simulink model "Iterative_Inverse_Kinematics"  (R2024a)
settings: Solver=ode4  StartTime=0.0  StopTime=inf  FixedStep=1/500  RelTol=1e-3  EnableMultiTasking=on
InitFcn:
  | home = [0.45; 0; 0.49];
  | default_w = [0.25; 0.25; 0.25];
  | default_a = [0.00; 0.375; 0.2];
  | A = [ 0.25; 0.25; 0.1];
  | B = [ 0.25; 0.50; 0.1];
  | C = [-0.25; 0.50; 0.1];
  | D = [-0.25; 0.25; 0.1];
  | 
  | waypoints_welding = [default_w, A, B, C, D, A]' ;
  | waypoints_assembly = [default_a, A, default_a, B, default_a, C, default_a, D]' ;
  | 
  | waypoints = waypoints_welding;
undefined symbols (not defined in the file): HIL, qc_get_step_size
libraries: quarc_library x9, simulink x2
settings Model: SimulationMode=external  ExtModeTrigDuration=10000  Creator=fvranes  LastModifiedBy=mbohra
settings SolverCC: AlgebraicLoopSolver=TrustRegion  PositivePriorityOrder=on
settings DataIOCC: SaveOutput=off  SignalLogging=off  DSMLogging=off  SaveTime=off  ReturnWorkspaceOutputs=off
settings DebuggingCC: UnconnectedInputMsg=warning  UnconnectedOutputMsg=warning  UnconnectedLineMsg=warning  ArithmeticOperatorsInVariantConditions=warning
settings ModelReferenceCC: EnableRefExpFcnMdlSchedulingChecks=on
settings SFSimCC: SimUseLocalCustomCode=off  CustomCodeUndefinedFunction=UseInterfaceOnly
settings RTWCC: Description=QUARC Win64 Target Using Toolchain  SystemTargetFile=quarc_win64.tlc  TemplateMakefile=quarc_default_tmf  RTWUseLocalCustomCode=off  Toolchain=QUARC win64 | nmake (64-bit Windows)  BuildConfiguration=Faster Runs  GPUComputeCapability=3.5
settings CodeAppCC: StateflowObjectComments=on
settings STFCustomTargetCC: ConcurrentExecutionCompliant=on  SystemTargetFile=quarc_win64.tlc
settings GRTTargetCC: ParMdlRefBuildCompliant=off  CompOptLevelCompliant=off  CombineOutputUpdateFcns=off  MatFileLogging=off  CPPClassGenCompliant=off  GRTInterface=on  ExtMode=on  ExtModeMexFile=quarc_comm
settings ConfigComp: CovMetricSettings=dswe

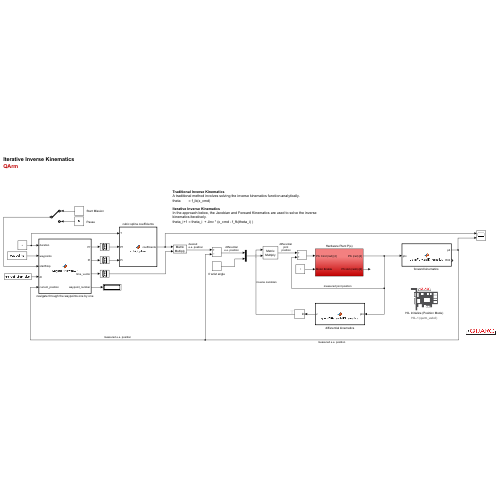
[thumbnail: Simulink's stored preview of the top-level diagram]
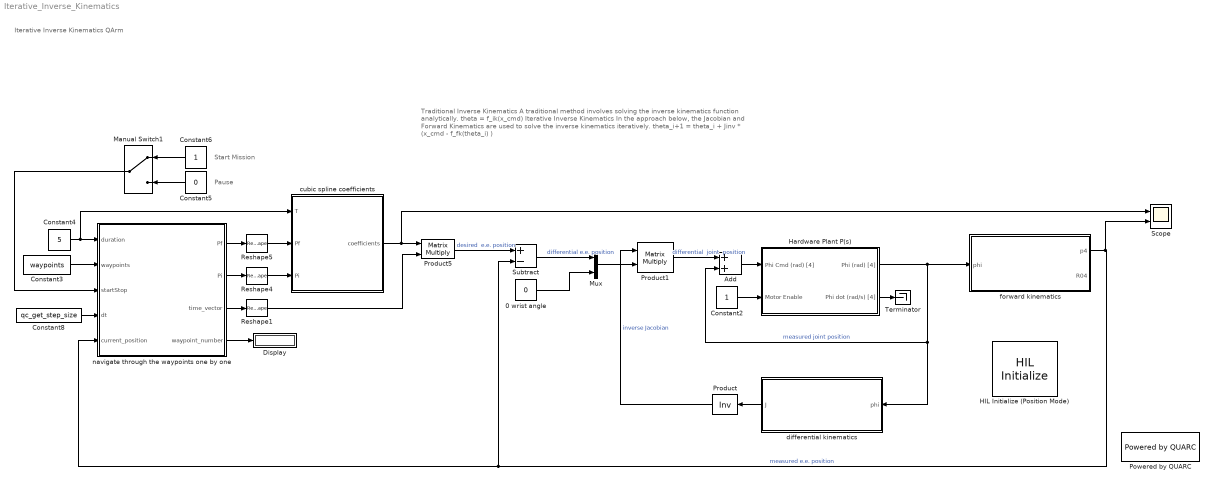
== system Iterative_Inverse_Kinematics ==
  note: Traditional Inverse Kinematics
      | A traditional method involves solving the inverse kinematics function analytically.
      | theta = f_ik(x_cmd)
      |
      | Iterative Inverse Kinematics
      | In the approach below, the Jacobian and Forward Kinematics are used to solve the inverse kinematics iteratively.
      | theta_i+1 = theta_i + Jinv * (x_cmd - f_fk(theta_i) )
  note: Iterative Inverse Kinematics
      | QArm
  note: Pause
  note: Start Mission
  0 wrist angle : Constant  Value=0
  Add : Sum
  Constant2 : Constant
  Constant3 : Constant  Value=waypoints  VectorParams1D=off
  Constant4 : Constant  Value=5
  Constant5 : Constant  Value=0
  Constant6 : Constant
  Constant8 : Constant  Value=qc_get_step_size
  Display : Display
  HIL Initialize (Position Mode) : quarc_library/Data Acquisition/Generic/Configuration/HIL Initialize  Priority=1  object_name=HIL-1  board_type=qarm_usb  board_number=0  board_options=j0_mode=0;j1_mode=0;j2_mode=0;j3_mode=0;gripper_mode=0;j0_profile_config=0;j0_profile_velocity=0;j0_profile_acceleration=0;j1_profile_config=0;j1_profile_velocity=0;j1_profile_acceleration=0;j2_profile_config=0;j2_profile_velocity=0;j2_profile_acceleration=0;j3_profile_config=0;j3_profile_velocity=0;j3_profile_acceleration=0;  exclusive=off  active=on  hardware_clocks=[0]  clock_modes=[]  initial_clock_frequencies=[]  set_clock_params_at_start=off  set_clock_params_at_switch_in=off  set_clock_frequencies_at_start=off  set_clock_frequencies_at_switch_in=off  analog_input_channels=[5:9]  analog_input_configurations=[]  analog_input_maximums=[]  analog_input_minimums=[]  set_analog_input_params_at_start=off  set_analog_input_params_at_switch_in=off  analog_output_channels=[]  analog_output_maximums=inf  analog_output_minimums=-inf  initial_analog_outputs=[0]  final_analog_outputs=[0]  watchdog_analog_outputs=[]  set_analog_output_params_at_start=off  set_analog_output_params_at_switch_in=off  set_analog_outputs_at_start=off  set_analog_outputs_at_switch_in=off  set_analog_outputs_at_terminate=off  set_analog_outputs_at_switch_out=off  set_analog_outputs_on_watchdog=off  digital_input_channels=[]  digital_output_channels=[]  digital_output_configuration=[]  initial_digital_outputs=[0]  final_digital_outputs=[0]  watchdog_digital_outputs=[0]  set_digital_output_params_at_start=off  set_digital_output_params_at_switch_in=off  set_digital_outputs_at_start=off  set_digital_outputs_at_switch_in=off  set_digital_outputs_at_terminate=off  set_digital_outputs_at_switch_out=off  set_digital_outputs_on_watchdog=off  encoder_channels=[]  quadrature=[]  encoder_filter_frequency=[]  initial_encoder_counts=[]  set_encoder_params_at_start=off  set_encoder_params_at_switch_in=off  set_encoder_counts_at_start=off  set_encoder_counts_at_switch_in=off  pwm_channels=[]  pwm_modes=[]  pwm_frequency=[]  pwm_configuration=[]  pwm_alignment=[]  pwm_polarity=[]  pwm_leading_deadband=[]  pwm_trailing_deadband=[]  initial_pwm_outputs=[]  final_pwm_outputs=[]  watchdog_pwm_outputs=[]  set_pwm_params_at_start=off  set_pwm_params_at_switch_in=off  set_pwm_outputs_at_start=off  set_pwm_outputs_at_switch_in=off  set_pwm_outputs_at_terminate=off  set_pwm_outputs_at_switch_out=off  set_pwm_outputs_on_watchdog=off  other_output_channels=[1000:1004 11000:11003 11005:11007]  initial_other_outputs=[zeros(1,9), ones(1,3)]  final_other_outputs=[zeros(1,9), ones(1,3)]  watchdog_other_outputs=zeros(1,12)  set_other_outputs_at_start=off  set_other_outputs_at_switch_in=off  set_other_outputs_at_terminate=off  set_other_outputs_at_switch_out=off  set_other_outputs_on_watchdog=off
  Hardware Plant P(s) : Subsystem
  Manual Switch1 : ManualSwitch
  Mux : Mux  Inputs=2
  Powered by QUARC : quarc_library/Logos/Powered by QUARC
  Product : Product  Inputs=/  Multiplication=Matrix(*)
  Product1 : Product  Multiplication=Matrix(*)
  Product5 : Product  Multiplication=Matrix(*)
  Reshape1 : Reshape  OutputDimensionality=Column vector (2-D)
  Reshape4 : Reshape  OutputDimensionality=Column vector (2-D)
  Reshape5 : Reshape  OutputDimensionality=Column vector (2-D)
  Scope : Scope  NumInputPorts=2
  Subtract : Sum  Inputs=+-
  Terminator : Terminator
  cubic spline coefficients : MATLAB Function  TreatAsAtomicUnit=on
  differential kinematics : MATLAB Function  TreatAsAtomicUnit=on
  "forward kinematics " : MATLAB Function  TreatAsAtomicUnit=on
  navigate through the waypoints one by one : MATLAB Function  TreatAsAtomicUnit=on
  wires:
  differential kinematics/1(J) -> Product/1
  Hardware Plant P(s)/1(Phi (rad) [4]) -> differential kinematics/1(phi), Add/2, "forward kinematics "/1(phi)  "measured joint position"
  "forward kinematics "/1(p4) -> Scope/2, navigate through the waypoints one by one/5(current_position), Subtract/2  "measured e.e. position"
  Product5/1 -> Subtract/1  "desired  e.e. position"
  Subtract/1 -> Mux/1  "differential e.e. position"
  Product/1 -> Product1/1  "inverse Jacobian"
  0 wrist angle/1 -> Mux/2
  Mux/1 -> Product1/2
  Product1/1 -> Add/1  "differential  joint  position"
  Add/1 -> Hardware Plant P(s)/1(Phi Cmd (rad) [4])
  Constant2/1 -> Hardware Plant P(s)/2(Motor Enable)
  Hardware Plant P(s)/2(Phi dot (rad/s) [4]) -> Terminator/1
  Reshape5/1 -> cubic spline coefficients/2(Pf)
  Constant5/1 -> Manual Switch1/2
  navigate through the waypoints one by one/3(time_vector) -> Reshape1/1
  Constant3/1 -> navigate through the waypoints one by one/2(waypoints)
  Reshape1/1 -> Product5/2
  Constant8/1 -> navigate through the waypoints one by one/4(dt)
  Constant4/1 -> cubic spline coefficients/1(T), navigate through the waypoints one by one/1(duration)
  navigate through the waypoints one by one/1(Pf) -> Reshape5/1
  Manual Switch1/1 -> navigate through the waypoints one by one/3(startStop)
  navigate through the waypoints one by one/2(Pi) -> Reshape4/1
  cubic spline coefficients/1(coefficients) -> Scope/1, Product5/1
  Constant6/1 -> Manual Switch1/1
  navigate through the waypoints one by one/4(waypoint_number) -> Display/1
  Reshape4/1 -> cubic spline coefficients/3(Pi)

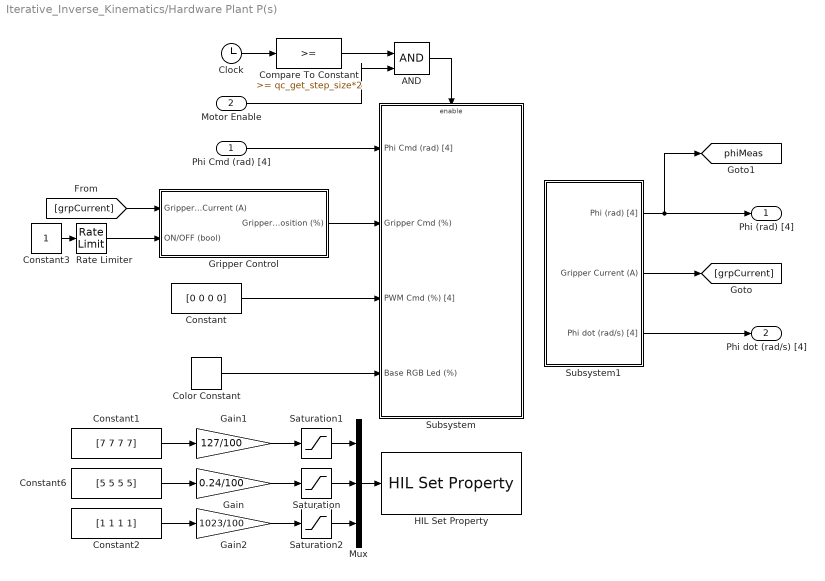
== system Iterative_Inverse_Kinematics/Hardware Plant P(s) ==
  Phi Cmd (rad) [4] : Inport
  Motor Enable : Inport  Port=2
  AND : Logic  IconShape=distinctive  AllPortsSameDT=off  OutDataTypeStr=boolean
  Clock : Clock
  Color Constant : quarc_library/Sources/Signals/Color Constant  color=[0.71765 0.27451 1]
      settings: SourceProductName=QUARC Targets
  Compare To Constant : simulink/Logic and Bit Operations/Compare To Constant  relop=>=  const=qc_get_step_size*2  OutDataTypeStr=boolean
  Constant : Constant  Value=[0 0 0 0]
  Constant1 : Constant  Value=[7 7 7 7]
  Constant2 : Constant  Value=[1 1 1 1]
  Constant3 : Constant
  Constant6 : Constant  Value=[5 5 5 5]
  Gain : Gain  Gain=0.24/100
  Gain1 : Gain  Gain=127/100
  Gain2 : Gain  Gain=1023/100
  Gripper Control : Subsystem
  HIL Set Property : quarc_library/Data Acquisition/Generic/Configuration/HIL Set Property  object_name=HIL-1  property_type=2  property_codes=[128:131, 133:136, 138:141]  property_source=2  property_value_num=0  set_at_start=on  sample_time=-1  active=off
      settings: AttributesFormatString=(%<object_name>)  SourceProductName=QUARC Targets
  Mux : Mux  Inputs=3
  Rate Limiter : RateLimiter  SampleTimeMode=inherited
  Saturation : Saturate  UpperLimit=0.24  LowerLimit=0
  Saturation1 : Saturate  UpperLimit=127  LowerLimit=0
  Saturation2 : Saturate  UpperLimit=1023  LowerLimit=0
  Subsystem : Subsystem
  Subsystem1 : Subsystem
  Phi (rad) [4] : Outport  VectorParamsAs1DForOutWhenUnconnected=off
  Phi dot (rad/s) [4] : Outport  Port=2  VectorParamsAs1DForOutWhenUnconnected=off
  tag scope: phiMeas=global
  wires:
  [grpCurrent] -> Gripper Control/1(Gripper Current (A))
  Phi Cmd (rad) [4]/1 -> Subsystem/1(Phi Cmd (rad) [4])
  Gripper Control/1(Gripper Position (%)) -> Subsystem/2(Gripper Cmd (%))
  Constant/1 -> Subsystem/3(PWM Cmd (%) [4])
  Compare To Constant/1 -> AND/1
  Clock/1 -> Compare To Constant/1
  Subsystem1/1(Phi (rad) [4]) -> [phiMeas], Phi (rad) [4]/1
  Subsystem1/3(Phi dot (rad/s) [4]) -> Phi dot (rad/s) [4]/1
  Subsystem1/2(Gripper Current (A)) -> [grpCurrent]
  Constant6/1 -> Gain/1
  Saturation/1 -> Mux/2
  Gain/1 -> Saturation/1
  Mux/1 -> HIL Set Property/1
  Gain1/1 -> Saturation1/1
  Constant1/1 -> Gain1/1
  Constant2/1 -> Gain2/1
  Gain2/1 -> Saturation2/1
  Saturation2/1 -> Mux/3
  Saturation1/1 -> Mux/1
  AND/1 -> Subsystem/Enable
  Motor Enable/1 -> AND/2
  Color Constant/1 -> Subsystem/4(Base RGB Led (%))
  Constant3/1 -> Rate Limiter/1
  Rate Limiter/1 -> Gripper Control/2(ON/OFF (bool))

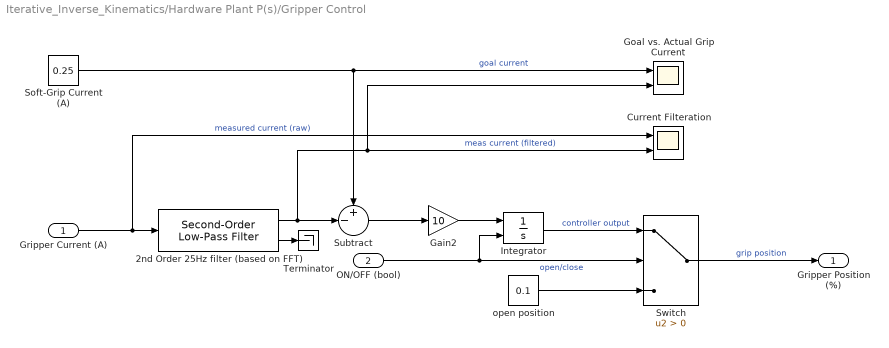
== system Iterative_Inverse_Kinematics/Hardware Plant P(s)/Gripper Control ==
  Gripper Current (A) : Inport
  ON/OFF (bool) : Inport  Port=2
  2nd Order 25Hz filter (based on FFT) : quarc_library/Continuous/Second-Order Low-Pass Filter  params_source=Internal (dialog parameters)  input_width=25*2*pi  input_zeta=1  input_init=0
  Current Filteration : Scope  NumInputPorts=2
  Gain2 : Gain  Gain=10
  Goal vs. Actual Grip Current : Scope  NumInputPorts=2
  Integrator : Integrator  ExternalReset=either  InitialCondition=0.1  LimitOutput=on  UpperSaturationLimit=0.9  LowerSaturationLimit=0.1
  Soft-Grip Current (A) : Constant  Value=0.25
  Subtract : Sum  Inputs=+-|
  Switch : Switch  Criteria=u2 > Threshold  SaturateOnIntegerOverflow=off  InputSameDT=off
  Terminator : Terminator
  open position : Constant  Value=0.1
  Gripper Position (%) : Outport  VectorParamsAs1DForOutWhenUnconnected=off
  wires:
  Gripper Current (A)/1 -> 2nd Order 25Hz filter (based on FFT)/1, Current Filteration/1  "measured current (raw)"
  ON/OFF (bool)/1 -> Switch/2, Integrator/2  "open/close"
  open position/1 -> Switch/3
  Switch/1 -> Gripper Position (%)/1  "grip position"
  Soft-Grip Current (A)/1 -> Subtract/1, Goal vs. Actual Grip Current/1  "goal current"
  2nd Order 25Hz filter (based on FFT)/1 -> Subtract/2, Current Filteration/2, Goal vs. Actual Grip Current/2  "meas current (filtered)"
  Subtract/1 -> Gain2/1
  Integrator/1 -> Switch/1  "controller output"
  Gain2/1 -> Integrator/1
  2nd Order 25Hz filter (based on FFT)/2 -> Terminator/1

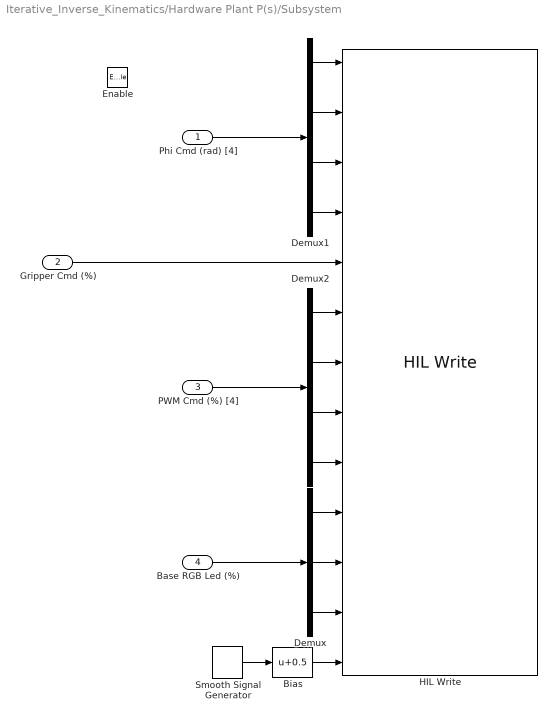
== system Iterative_Inverse_Kinematics/Hardware Plant P(s)/Subsystem ==
  Phi Cmd (rad) [4] : Inport
  Gripper Cmd (%) : Inport  Port=2
  PWM Cmd (%) [4] : Inport  Port=3
  Base RGB Led (%) : Inport  Port=4
  Enable : EnablePort
  Bias : Bias  Bias=0.5  SaturateOnIntegerOverflow=off
  Demux : Demux  Outputs=3
  Demux1 : Demux
  Demux2 : Demux
  HIL Write : quarc_library/Data Acquisition/Generic/Immediate I//O/HIL Write  object_name=HIL-1  analog_channels=[]  pwm_channels=[]  digital_channels=[]  other_channels=[1000:1004 11000:11003 11005:11008]  sample_time=-1  active=on  vector_input=off
  Smooth Signal Generator : quarc_library/Sources/Signals/Smooth Signal Generator  signal_type=Sine  source=Internal (dialog parameters)  amplitude=0.5  frequency=0.5  initial_phase=0  sample_time=qc_get_step_size  output_cos=off
      settings: SourceProductName=QUARC Targets
  wires:
  Demux2/3 -> HIL Write/8
  Demux2/4 -> HIL Write/9
  Demux1/1 -> HIL Write/1
  Demux2/1 -> HIL Write/6
  Demux2/2 -> HIL Write/7
  PWM Cmd (%) [4]/1 -> Demux2/1
  Demux1/3 -> HIL Write/3
  Demux/3 -> HIL Write/12
  Smooth Signal Generator/1 -> Bias/1
  Phi Cmd (rad) [4]/1 -> Demux1/1
  Bias/1 -> HIL Write/13
  Gripper Cmd (%)/1 -> HIL Write/5
  Demux1/2 -> HIL Write/2
  Demux/1 -> HIL Write/10
  Demux/2 -> HIL Write/11
  Base RGB Led (%)/1 -> Demux/1
  Demux1/4 -> HIL Write/4

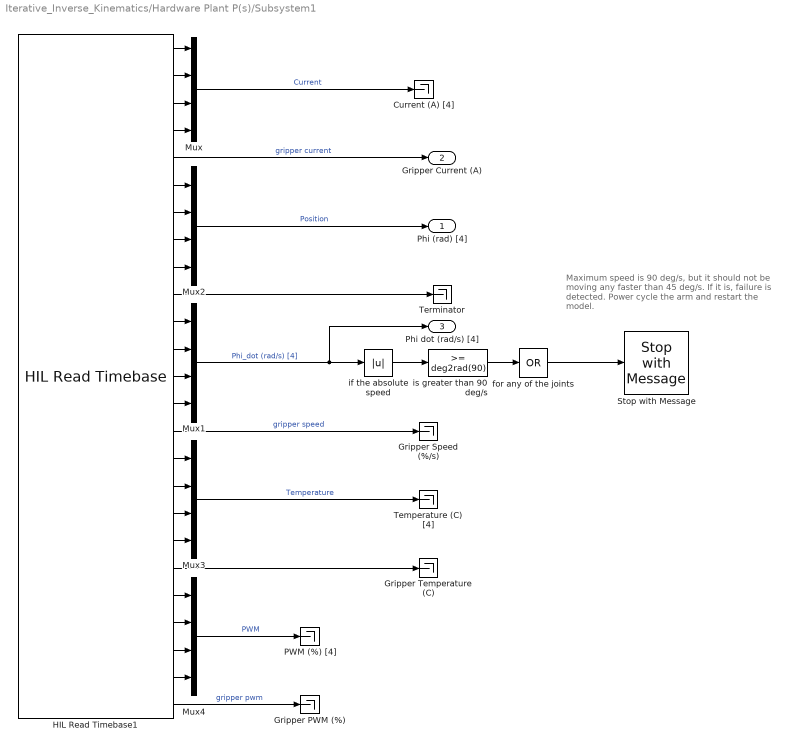
== system Iterative_Inverse_Kinematics/Hardware Plant P(s)/Subsystem1 ==
  note: Maximum speed is 90 deg/s, but it should not
      | be moving any faster than 45 deg/s. If it is,
      | failure is detected. Power cycle the arm and
      | restart the model.
  Current (A) [4] : Terminator
  Gripper PWM (%) : Terminator
  Gripper Speed (%/s) : Terminator
  Gripper Temperature (C) : Terminator
  HIL Read Timebase1 : quarc_library/Data Acquisition/Generic/Timebases/HIL Read Timebase  object_name=HIL-1  clock=0  analog_channels=[5:9]  encoder_channels=[]  digital_channels=[]  other_channels=[1000:1004 3000:3004 10000:10004 11000:11004]  active=on  vector_output=off  data_type_mode=Inherit via back propagation  encoder_data_type=double  digital_data_type=boolean  overflow_mode=Error on overflow  samples_in_buffer=max(ceil(1/qc_get_step_size), 1)
  Mux{,1..4} (5 alike) : Mux
  PWM (%) [4] : Terminator
  Stop with Message : quarc_library/Sinks/Error Handling/Stop with Message  message_type=Fixed error message  message_icon=Error  message=Arm moving close to maximum speed.
  Temperature (C) [4] : Terminator
  Terminator : Terminator
  for any of the joints : Logic  Operator=OR  Inputs=1  IconShape=distinctive  AllPortsSameDT=off  OutDataTypeStr=boolean
  if the absolute speed : Abs  SaturateOnIntegerOverflow=off
  is greater than 90 deg/s : simulink/Logic and Bit Operations/Compare To Constant  relop=>=  const=deg2rad(90)  OutDataTypeStr=boolean
  Phi (rad) [4] : Outport  VectorParamsAs1DForOutWhenUnconnected=off
  Gripper Current (A) : Outport  Port=2  VectorParamsAs1DForOutWhenUnconnected=off
  Phi dot (rad/s) [4] : Outport  Port=3  VectorParamsAs1DForOutWhenUnconnected=off
  wires:
  HIL Read Timebase1/15 -> Gripper Speed (%/s)/1  "gripper speed"
  Mux1/1 -> Phi dot (rad/s) [4]/1, if the absolute speed/1  "Phi_dot (rad/s) [4]"
  Mux2/1 -> Phi (rad) [4]/1  "Position"
  HIL Read Timebase1/9 -> Mux2/4
  Mux3/1 -> Temperature (C) [4]/1  "Temperature"
  HIL Read Timebase1/25 -> Gripper PWM (%)/1  "gripper pwm"
  HIL Read Timebase1/3 -> Mux/3
  HIL Read Timebase1/23 -> Mux4/3
  HIL Read Timebase1/13 -> Mux1/3
  Mux4/1 -> PWM (%) [4]/1  "PWM"
  HIL Read Timebase1/18 -> Mux3/3
  HIL Read Timebase1/17 -> Mux3/2
  HIL Read Timebase1/22 -> Mux4/2
  HIL Read Timebase1/20 -> Gripper Temperature (C)/1
  HIL Read Timebase1/21 -> Mux4/1
  HIL Read Timebase1/2 -> Mux/2
  HIL Read Timebase1/1 -> Mux/1
  HIL Read Timebase1/10 -> Terminator/1
  HIL Read Timebase1/24 -> Mux4/4
  HIL Read Timebase1/7 -> Mux2/2
  Mux/1 -> Current (A) [4]/1  "Current"
  HIL Read Timebase1/8 -> Mux2/3
  HIL Read Timebase1/19 -> Mux3/4
  HIL Read Timebase1/6 -> Mux2/1
  HIL Read Timebase1/14 -> Mux1/4
  HIL Read Timebase1/11 -> Mux1/1
  HIL Read Timebase1/5 -> Gripper Current (A)/1  "gripper current"
  HIL Read Timebase1/4 -> Mux/4
  HIL Read Timebase1/12 -> Mux1/2
  HIL Read Timebase1/16 -> Mux3/1
  if the absolute speed/1 -> is greater than 90 deg/s/1
  is greater than 90 deg/s/1 -> for any of the joints/1
  for any of the joints/1 -> Stop with Message/1

== matlab function Iterative_Inverse_Kinematics/differential kinematics ==
  data: phi input; J output
function J   = qarmDifferentialKinematics(phi)

%% QUANSER_ARM_FDK
% v 1.0 - 13th August 2020

% REFERENCE: 
% Chapter 5. Velocity Kinematics
% Robot Dynamics and Control 
% Spong, Vidyasagar
% 1989

% INPUTS:
% phi     : Alternate joint angles vector 4 x 1

% OUTPUTS:
% p4      : End-effector frame {4} position vector expressed in base frame {0}
% R04     : rotation matrix from end-effector frame {4} to base frame {0}

%% Manipulator parameters:
L1 = 0.1400;
L2 = 0.3500;
L3 = 0.0500;
L4 = 0.2500;
L5 = 0.1500;

%% Alternate parameters
l1 = L1;
l2 = sqrt(L2^2 + L3^2);
l3 = L4 + L5;
beta = atan(L3/L2);

%% From phi space to theta space 
theta = phi;
theta(1) = phi(1);
theta(2) = phi(2) + beta - pi/2;
theta(3) = phi(3) - beta;
theta(4) = phi(4);

%% Jacobian term definition:

J = eye(4);
J(1,1) = - l2*sin(theta(1))*cos(theta(2)) + l3*sin(theta(1))*sin(theta(2)+theta(3)); 
J(1,2) = - l2*cos(theta(1))*sin(theta(2)) - l3*cos(theta(1))*cos(theta(2)+theta(3)); 
J(1,3) = - l3*cos(theta(1))*cos(theta(2)+theta(3)); 
J(1,4) = 0;
J(2,1) =   l2*cos(theta(1))*cos(theta(2)) - l3*cos(theta(1))*sin(theta(2)+theta(3)); 
J(2,2) = - l2*sin(theta(1))*sin(theta(2)) - l3*sin(theta(1))*cos(theta(2)+theta(3)); 
J(2,3) = - l3*sin(theta(1))*cos(theta(2)+theta(3));
J(2,4) = 0;
J(3,1) = 0; 
J(3,2) = - l2*cos(theta(2)) + l3*sin(theta(2)+theta(3)); 
J(3,3) =   l3*sin(theta(2)+theta(3));
J(3,4) = 0;
J(4,1) = 0;
J(4,2) = 0;
J(4,3) = 0;
J(4,4) = 1;

end

== matlab function Iterative_Inverse_Kinematics/cubic spline coefficients ==
  data: T input; coefficients output; Pf input; Pi input
function coefficients = cubicSpline(T, Pf, Pi)

% Cubic spline coefficients for X, Y and Z (coloumns)
a0 = [                     Pi(1,1);                      Pi(2,1);                     Pi(3,1)];
a1 = [                           0;                            0;                            0];
a2 = [ 3*(Pf(1,1) - Pi(1,1))/(T^2);  3*(Pf(2,1) - Pi(2,1))/(T^2);  3*(Pf(3,1) - Pi(3,1))/(T^2)];
a3 = [-2*(Pf(1,1) - Pi(1,1))/(T^3); -2*(Pf(2,1) - Pi(2,1))/(T^3); -2*(Pf(3,1) - Pi(3,1))/(T^3)];

% Output coefficients as a 3 x 4 matrix (1 row each for x, y and z)
coefficients = [a0, a1, a2, a3];

== matlab function Iterative_Inverse_Kinematics/navigate through the waypoints one by one ==
  data: duration input; waypoints input; Pf output; startStop input; dt input; current_position input; Pi output; time_vector output; waypoint_number output
function [Pf, Pi, time_vector, waypoint_number] = waypointNavigator(duration, waypoints, startStop, dt, current_position)

%% Initialization of internal variables
% Use persistent variables to track states across multiple iterations, and 
% define them on first call
persistent initial final next t
    if isempty(initial) || isempty(final)
        initial = current_position;
        final = current_position;
    end
    if isempty(next)
        next = 0;
    end
    if isempty(t)
        t = 0;
    end
    
% Find the number of waypoints in total    
[num_waypoints, ~] = size(waypoints);

%% Timing between the waypoints
% Ensure timer remains between 0 and duration
t_mod = mod(t, duration);

% Raise the flag if the timer resets to 0 (proceed to the next waypoint)
flag = t_mod < t;

%% Updating waypoints
if flag
    % proceed to the next waypoint
    next = next + 1;
    
    % cycle back to the first waypoint after the last one
    if next > num_waypoints
        next = 1;
    end

    % set the final and inital internal variables 
    final = waypoints(next, :)';
    initial = current_position;
end

%% Update the internal timer t
t = t_mod;
if startStop
    t = t + dt;
end

%% Set the outputs
waypoint_number = next; 
time_vector = [1; t; t^2; t^3];
Pf = final;
Pi = initial;

== matlab function Iterative_Inverse_Kinematics/forward kinematics  ==
  data: phi input; p4 output; R04 output
function [p4, R04] = qarmForwardKinematics(phi)

%% QUANSER_ARM_FPK
% v 4.0 - 4th June 2020

% REFERENCE: 
% Chapter 3. Forward Kinematics
% Robot Dynamics and Control 
% Spong, Vidyasagar
% 1989

% INPUTS:
% phi     : Alternate joint angles vector 4 x 1

% OUTPUTS:
% p4      : End-effector frame {4} position vector expressed in base frame {0}
% R04     : rotation matrix from end-effector frame {4} to base frame {0}

%% Manipulator parameters:
L1 = 0.1400;
L2 = 0.3500;
L3 = 0.0500;
L4 = 0.2500;
L5 = 0.1500;

%% Alternate parameters
l1 = L1;
l2 = sqrt(L2^2 + L3^2);
l3 = L4 + L5;
beta = atan(L3/L2);

%% From phi space to theta space 
theta = phi;
theta(1) = phi(1);
theta(2) = phi(2) + beta - pi/2;
theta(3) = phi(3) - beta;
theta(4) = phi(4);

%% Transformation matrices for all frames:

% T{i-1}{i} = quanser_arm_DH(  a, alpha,  d,     theta );
        T01 = quanser_arm_DH(  0, -pi/2, l1,  theta(1) );
        T12 = quanser_arm_DH( l2,     0,  0,  theta(2) );
        T23 = quanser_arm_DH(  0, -pi/2,  0,  theta(3) );
        T34 = quanser_arm_DH(  0,     0, l3,  theta(4) );

        T02 = T01*T12;
        T03 = T02*T23;
        T04 = T03*T34;

%% Position of end-effector Transformation

% Extract the Position vector 
% p1   = T01(1:3,4);
% p2   = T02(1:3,4);
% p3   = T03(1:3,4);
p4   = T04(1:3,4);

% Extract the Rotation matrix
% R01 = T01(1:3,1:3);
% R02 = T02(1:3,1:3);
% R03 = T03(1:3,1:3);
R04 = T04(1:3,1:3);

end

function T = quanser_arm_DH(a,alpha,d,theta)

%% QUANSER_ARM_DH
% v 1.0 - 26th March 2019

% REFERENCE: 
% Chapter 3. Forward and Inverse Kinematics
% Robot Modeling and Control 
% Spong, Hutchinson, Vidyasagar
% 2006

% INPUTS:
% a       :   translation  : along : x_{i}   : from : z_{i-1} : to : z_{i}
% alpha   :      rotation  : about : x_{i}   : from : z_{i-1} : to : z_{i}
% d       :   translation  : along : z_{i-1} : from : x_{i-1} : to : x_{i}
% theta   :      rotation  : about : z_{i-1} : from : x_{i-1} : to : x_{i}
% NOTE: Standard DH Parameters

% OUTPUTS:
% T       : transformation                   : from :     {i} : to : {i-1}

%%
% Rotation Transformation about z axis by theta
T_R_z = [cos(theta) -sin(theta) 0 0;
         sin(theta)  cos(theta) 0 0;
                  0           0 1 0;
                  0           0 0 1];
     
% Translation Transformation along z axis by d
T_T_z = [1 0 0 0;
         0 1 0 0;
         0 0 1 d;
         0 0 0 1];

% Translation Transformation along x axis by a
T_T_x = [1 0 0 a;
         0 1 0 0;
         0 0 1 0;
         0 0 0 1];

% Rotation Transformation about x axis by alpha
T_R_x = [1          0           0 0;
         0 cos(alpha) -sin(alpha) 0;
         0 sin(alpha)  cos(alpha) 0;
         0          0           0 1];

% For a transformation FROM frame {i} TO frame {i-1}: A
T = T_R_z*T_T_z*T_T_x*T_R_x;

end
